simulink model "Test_DMP"  (R2018a)
settings: Solver=VariableStepAuto  StartTime=0.0  StopTime=2*tau  RelTol=1e-3
values from neighbouring files (symbols this model uses):
  Am = repmat(Am,1,6/length(Am))    [CostFCN.m]    (also in optimizeRobotMotion_openLoop.m; pFinal_runSim.m; simWalker_constraint.m)
  dt = .01    (= 0.01)    [Trajectory.m]    (also in rcp.m = 0.001)
  init_pos = Am'.*init_pos    [CostFCN.m]    (also in optimizeRobotMotion_openLoop.m; pFinal_runSim.m; simWalker_constraint.m)
  init_vel = Am'.*init_vel    [CostFCN.m]    (also in optimizeRobotMotion_openLoop.m; pFinal_runSim.m; simWalker_constraint.m)
  tau = params(1,2)    [CostFCN.m]    (also in Test_params.m = tau_nom; Trajectory.m = (2*pi)/omega; optimizeRobotMotion_openLoop.m = pFinal(1,2); pFinal_runSim.m = pFinal(1,2))
  Ym = Ym.*Am    [CostFCN.m]    (also in optimizeRobotMotion_openLoop.m; pFinal_runSim.m; simWalker_constraint.m)
undefined symbols (not defined in the file or in its folder): init_pos2, init_vel2, W, W2, Ym2
libraries: simulink_extras x6
(part 2 of 2)

== matlab function Test_DMP/DMP Generation2/DMP+Initiation2 ==
  data: t input; dt input; DMP_rev output; Y input
function DMP_rev = fcn(t, dt, Y)

yy = 0;

for j = 1:6
    
    %% Knee Trajectories saturation
    if j==2 || j==5
        if Y(j)<0
            Y(j) = 0;
        end
    end
    
    %% Smoothening of the Hip Trajectories Notches
%     if t>156*dt && t<174*dt
%         
%         if j==1 || j==4
%             if t == 156*dt
%                 yy = Y(j);
%             end
%             
%             Y(j)=yy+(Y(j)-yy)*(t/dt-156)'/17;
%         end
%     end
    
    %% Set up the initial trajectory bridging the double-stance phase to the onset of the DMP Trajectory
    if t<=.01
        if j==1
            Y(j) = 0;
        elseif j==2
            Y(j) = 0;
        elseif j==4
            Y(j) = 0;
        elseif  j==3 || j==6
            Y(j) = 0;
        elseif j==5
            Y(j) = 0;
        end
    elseif t<=.45
        if j==1
            Y(j) = -22.09*t/.45;
        elseif j==2
            Y(j) = 5.86*t/.45;
        elseif j==4     % right hip in orange
            Y(j) = 4.7*t/.45;
        elseif  j==3 || j==6    % 6: right ankle in yellow
            Y(j) = 0;
        elseif j==5     % right knee in blue
            Y(j) = -(6/.2^2)*(t-.2).^2+3;
            if Y(j)<0
                Y(j)=0;
            end

        end
        
    elseif t>.45 && t<=.475
        Y(4)=4.7-(t-.45)/.025*.75;
        
    
        
    end
    
    %% The final revised DMP
    DMP_rev = Y(end:-1:1);
end

== matlab function Test_DMP/DMP Generation2/DMP+Initiation3 ==
  data: t input; dt input; DMP_rev output; Y input
function DMP_rev = fcn(t, dt, Y)

yy = 0;

for j = 1:6
    
    %% Knee Trajectories saturation
    if j==2 || j==5
        if Y(j)<0
            Y(j) = 0;
        end
    end
    
    %% Smoothening of the Hip Trajectories Notches
%     if t>156*dt && t<174*dt
%         
%         if j==1 || j==4
%             if t == 156*dt
%                 yy = Y(j);
%             end
%             
%             Y(j)=yy+(Y(j)-yy)*(t/dt-156)'/17;
%         end
%     end
    
    %% Set up the initial trajectory bridging the double-stance phase to the onset of the DMP Trajectory
    
    if t<=.0001
        if j==1
            Y(j) = 0;
        elseif j==2
            Y(j) = 0;
        elseif j==4
            Y(j) = 0;
        elseif  j==3 || j==6
            Y(j) = 0;
        elseif j==5
            Y(j) = 0;
        end
        
    elseif t<.59
        if j==1
            Y(j) = -22.09*t/.59;
        elseif j==2
            Y(j) = 5.86*t/.59;
        elseif j==4
            Y(j) = 8.66*t/.59;
        elseif  j==3 || j==6
            Y(j) = 0;
        elseif j==5
            Y(j) = -(6/.29^2)*(t-.29).^2+3;
        end
               
    end
    
    %% The final revised DMP
    DMP_rev = Y(end:-1:1);
end

== matlab function Test_DMP/DMP Generation2/DMP+Initiation4 ==
  data: t input; init_pos input; DMP_rev output; Y input
function DMP_rev = fcn(t, init_pos, Y)

yy = 0;

for j = 1:6
    
    %% Knee Trajectories saturation
    if j==2 || j==5
        if Y(j)<0
            Y(j) = 0;
        end
    end
    
    %% Smoothening of the Hip Trajectories Notches
%     if t>156*dt && t<174*dt
%         
%         if j==1 || j==4
%             if t == 156*dt
%                 yy = Y(j);
%             end
%             
%             Y(j)=yy+(Y(j)-yy)*(t/dt-156)'/17;
%         end
%     end
    
    %% Set up the initial trajectory bridging the double-stance phase to the onset of the DMP Trajectory
%     if t<=.01
%         if j==1
%             Y(j) = 0;
%         elseif j==2
%             Y(j) = 0;
%         elseif j==4
%             Y(j) = 0;
%         elseif  j==3 || j==6
%             Y(j) = 0;
%         elseif j==5
%             Y(j) = 0;
%         end
%         
%     %%%    
% %     elseif t<=.59
% %         if j==1
% %             Y(j) = -22.09*t/.59;
% %         elseif j==2
% %             Y(j) = 5.86*t/.59;
% %         elseif j==4     % right hip in orange
% %             Y(j) = -4.7*t/.59;
% %         elseif  j==3 || j==6    % 6: right ankle in yellow
% %             Y(j) = 0;
% %         elseif j==5     % right knee in blue
% %             Y(j) = -(6/.29^2)*(t-.29).^2+3;
% %             if Y(j)<0
% %                 Y(j)=0;
% %             end
% %             
% % 
% %         end
%        %%%% 
% %     elseif t>.45 && t<=.475
% %         Y(4)=4.7-(t-.45)/.025*.75;
%     %%%%    
%     elseif t<=.67
%         if j==1
%             Y(j) = +23/(.39)^2*(t-.39).^2-23;
%         elseif j==4
%             Y(j) = 5*t/.65;
%         elseif  j==3   % 6: right ankle in yellow
%             Y(j) = -0*t/.65;
%         elseif  j==6   % 6: right ankle in yellow
%             Y(j) = 0;
%         elseif j==2
%             Y(j)= 14*t/.6;
%             
%         elseif j==5     % right knee in blue
%             Y(j) = -(10/.29^2)*(t-.29).^2+10;
%             if Y(j)<0
%                 Y(j)=0;
%             end
%             
% 
%         end
%     %%%%%    
%     end
    
    %% The final revised DMP
    DMP_rev = Y(end:-1:1);
end

== matlab function Test_DMP/DMP Generation2/Forcing_Term1 ==
  data: f output; PSI input; W input; Amp input
function f = fcn(PSI,W,Amp)

f = zeros(1,6);

for i=1:6
%     amp = Amp(i);
    w   = W(:,i);
    psi = PSI(:,i);
    
    f(i)            = sum(w.*psi)/sum(psi+1.e-10) * Amp;
    
end
end

== matlab function Test_DMP/DMP Generation2/Forcing_Term2 ==
  data: f output; PSI input; W input; Amp input
function f = fcn(PSI,W,Amp)

f = zeros(1,6);

for i=1:6
%     amp = Amp(i);
    w   = W(:,i);
    psi = PSI(:,i);
    
    f(i)            = sum(w.*psi)/sum(psi+1.e-10) * Amp;
    
end
end

== matlab function Test_DMP/DMP Generation2/Gaussian_fun1 ==
  data: PSI output; Phi input
function PSI = fcn(Phi)

n_rfs  = 50;    % number of kernel functions

% the time constants for chosen for critical damping

c       = 2*pi*(1/n_rfs:1/n_rfs:1)';
D       = ones(n_rfs,1)*.1*n_rfs^2;

PSI = zeros(n_rfs,6);

for i=1:6
    
    p = Phi;
    
    PSI(:,i) = exp(D.*(cos(p-c)-1));
    
end

== matlab function Test_DMP/DMP Generation2/Gaussian_fun2 ==
  data: PSI output; Phi input
function PSI = fcn(Phi)

n_rfs  = 100;    % number of kernel functions

% the time constants for chosen for critical damping

c       = 2*pi*(1/n_rfs:1/n_rfs:1)';
D       = ones(n_rfs,1)*.1*n_rfs^2;

PSI = zeros(n_rfs,6);

for i=1:6
    
    p = Phi;
    
    PSI(:,i) = exp(D.*(cos(p-c)-1));
    
end

== matlab function Test_DMP/DMP Generation2/Initial States ==
  data: tau input; pos_i output; init_pos input; init_vel input; z_i output
function [pos_i, z_i] = fcn(tau,init_pos,init_vel)

pos_i = zeros(6,1);
z_i   = zeros(6,1);
for i=1:6

    pos_i(i,1)   = init_pos(i,1);
    vel_i   = init_vel(i,1);
    z_i(i,1)     = vel_i*tau;
        
end
    
end
